simulink model "ej7"  (R2023a)
settings: Solver=ode23  StartTime=0.0  StopTime=5000  MaxStep=0.001  RelTol=1e-3
settings Model: Creator=santi  LastModifiedBy=santi

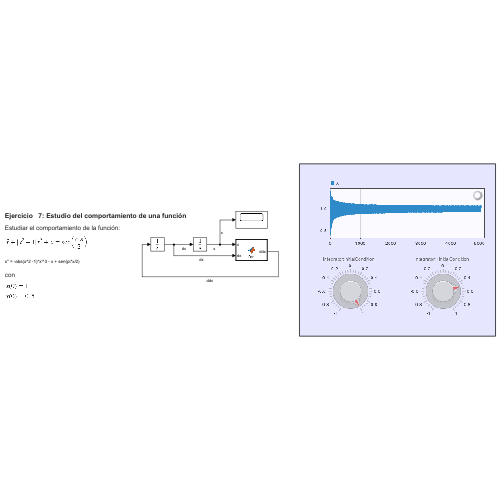
[thumbnail: Simulink's stored preview of the top-level diagram]
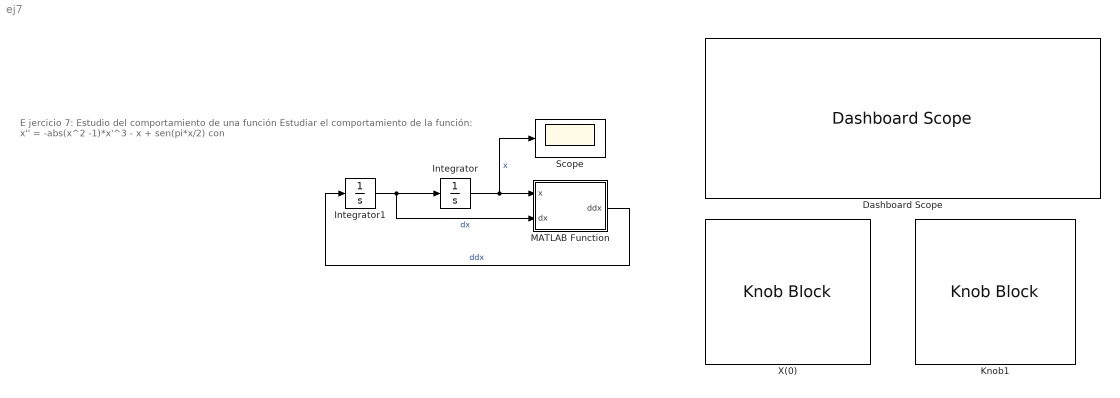
== system ej7 ==
  note: E jercicio 7: Estudio del comportamiento de una función
      | Estudiar el comportamiento de la función:
      |
      | x'' = -abs(x^2 -1)*x'^3 - x + sen(pi*x/2)
      | con
  Dashboard Scope : DashboardScope
  Integrator : Integrator  InitialCondition=1
  Integrator1 : Integrator  InitialCondition=0.5
  Knob1 : KnobBlock  ScaleMin=-1  ScaleMax=1
  MATLAB Function : MATLAB Function  TreatAsAtomicUnit=on
  Scope : Scope
  X(0) : KnobBlock  ScaleMin=-1  ScaleMax=1
  wires:
  Integrator1/1 -> Integrator/1, MATLAB Function/2(dx)  "dx"
  Integrator/1 -> Scope/1, MATLAB Function/1(x)  "x"
  MATLAB Function/1(ddx) -> Integrator1/1  "ddx"

== matlab function ej7/MATLAB Function ==
  data: x input; ddx output; dx input
function ddx = fcn(x, dx)

ddx = -abs(x^2 -1)*dx^3 - x + sin(pi*x/2);
